simulink model "A_CruiseControl"  (R2021b)
settings: Solver=VariableStepAuto  StartTime=0.0  StopTime=400  RelTol=1e-3
settings Model: Creator=vigne  LastModifiedBy=vigne

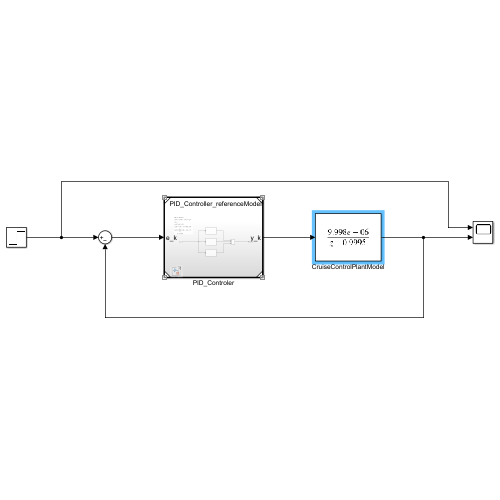
[thumbnail: Simulink's stored preview of the top-level diagram]
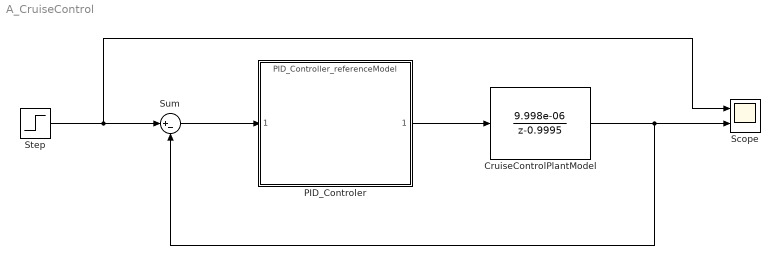
== system A_CruiseControl ==
  CruiseControlPlantModel : DiscreteTransferFcn  Numerator=[9.998e-06]  Denominator=[1 -0.9995]
  PID_Controler : ModelReference  ModelNameDialog=PID_Controller_referenceModel.slx  ModelReferenceVersion=1.6
  Scope : Scope  NumInputPorts=2
  Step : Step  After=1000  SampleTime=0
  Sum : Sum  Inputs=|+-
  wires:
  CruiseControlPlantModel/1 -> Sum/2, Scope/2
  Step/1 -> Scope/1, Sum/1
  Sum/1 -> PID_Controler/1
  PID_Controler/1 -> CruiseControlPlantModel/1
